simulink model "hw2_eserc_4_simulink_new"  (R2023b)
settings: Solver=FixedStepAuto  StartTime=0.0  StopTime=10  FixedStep=1/fs  RelTol=1e-3
undefined symbols (not defined in the file or in its folder): b, k1, k2
libraries: robotmobilelib x1
settings Model: Creator=ANDREA  LastModifiedBy=lalla

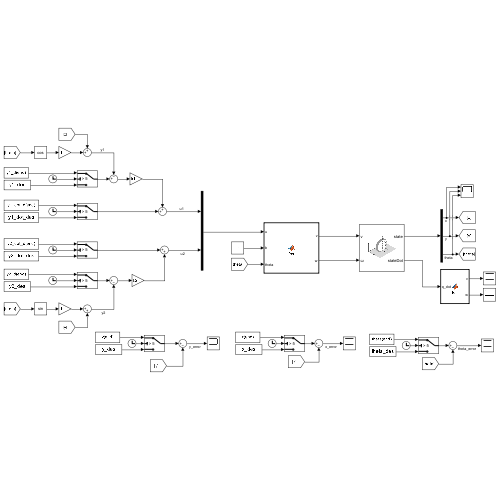
[thumbnail: Simulink's stored preview of the top-level diagram]
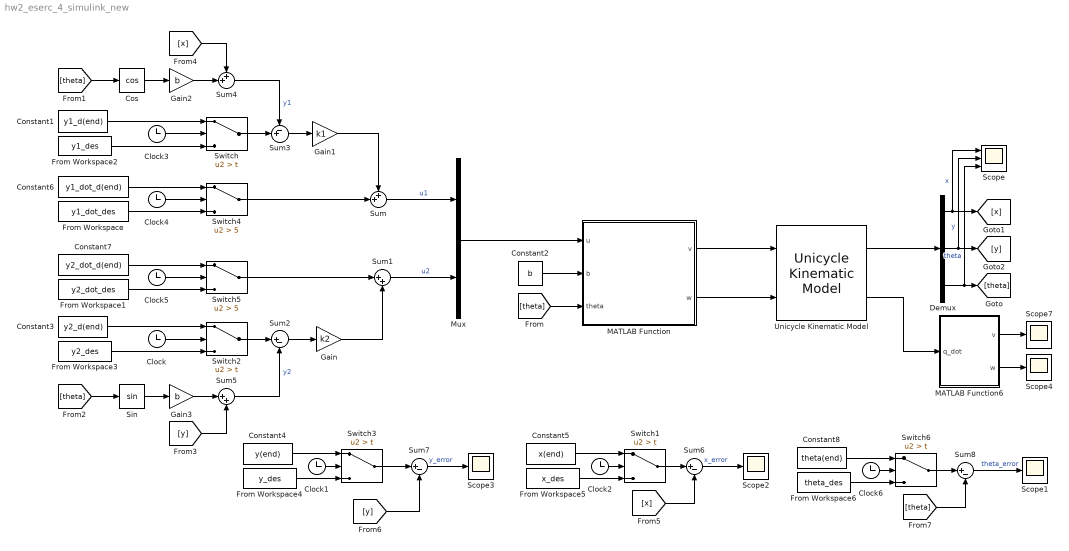
== system hw2_eserc_4_simulink_new ==
  Clock{,1..6} (7 alike) : Clock
  Constant1 : Constant  Value=y1_d(end)
  Constant2 : Constant  Value=b
  Constant3 : Constant  Value=y2_d(end)
  Constant4 : Constant  Value=y(end)
  Constant5 : Constant  Value=x(end)
  Constant6 : Constant  Value=y1_dot_d(end)
  Constant7 : Constant  Value=y2_dot_d(end)
  Constant8 : Constant  Value=theta(end)
  Cos : Trigonometry  Operator=cos
  Demux : Demux  Outputs=3
  From Workspace : FromWorkspace  VariableName=y1_dot_des
  From Workspace1 : FromWorkspace  VariableName=y2_dot_des
  From Workspace2 : FromWorkspace  VariableName=y1_des
  From Workspace3 : FromWorkspace  VariableName=y2_des
  From Workspace4 : FromWorkspace  VariableName=y_des
  From Workspace5 : FromWorkspace  VariableName=x_des
  From Workspace6 : FromWorkspace  VariableName=theta_des
  Gain : Gain  Gain=k2
  Gain1 : Gain  Gain=k1
  Gain2 : Gain  Gain=b
  Gain3 : Gain  Gain=b
  MATLAB Function : MATLAB Function  TreatAsAtomicUnit=on
  MATLAB Function6 : MATLAB Function  TreatAsAtomicUnit=on
  Mux : Mux  Inputs=2
  Scope : Scope  NumInputPorts=3
  Scope{1..4,7} (5 alike) : Scope
  Sin : Trigonometry
  Sum : Sum  Inputs=++|
  Sum1 : Sum  Inputs=|++
  Sum{2,6..8} (4 alike) : Sum  Inputs=|+-
  Sum3 : Sum  Inputs=-+|
  Sum4 : Sum  Inputs=++|
  Sum5 : Sum  Inputs=|++
  Switch{,1..3,6} (5 alike) : Switch  Criteria=u2 > Threshold  Threshold=t  SaturateOnIntegerOverflow=off  InputSameDT=off
  Switch4 : Switch  Criteria=u2 > Threshold  Threshold=5  SaturateOnIntegerOverflow=off  InputSameDT=off
  Switch5 : Switch  Criteria=u2 > Threshold  Threshold=5  SaturateOnIntegerOverflow=off  InputSameDT=off
  Unicycle Kinematic Model : robotmobilelib/Unicycle Kinematic Model  VehicleInputs=Vehicle Speed & Heading Angular Velocity  WheelRadius=b  WheelSpeedRange=[-Inf Inf]  InitialState=[0; 0; 0]  SimulateUsing=Interpreted execution
  wires:
  Unicycle Kinematic Model/1 -> Demux/1
  Gain/1 -> Sum1/2
  Sum3/1 -> Gain1/1
  Sum2/1 -> Gain/1
  Constant2/1 -> MATLAB Function/2(b)
  Cos/1 -> Gain2/1
  Sin/1 -> Gain3/1
  Demux/3 -> Scope/3, [theta]  "theta"
  [theta] -> MATLAB Function/3(theta)
  [theta] -> Cos/1
  [theta] -> Sin/1
  Gain2/1 -> Sum4/2
  Sum/1 -> Mux/1  "u1"
  Sum1/1 -> Mux/2  "u2"
  Mux/1 -> MATLAB Function/1(u)
  Demux/1 -> Scope/1, [x]  "x"
  Demux/2 -> Scope/2, [y]  "y"
  [x] -> Sum4/1
  Gain3/1 -> Sum5/1
  [y] -> Sum5/2
  MATLAB Function/2(w) -> Unicycle Kinematic Model/2
  MATLAB Function/1(v) -> Unicycle Kinematic Model/1
  Sum7/1 -> Scope3/1  "y_error"
  Sum6/1 -> Scope2/1  "x_error"
  Gain1/1 -> Sum/1
  Sum5/1 -> Sum2/2  "y2"
  Sum4/1 -> Sum3/1  "y1"
  [y] -> Sum7/2
  [x] -> Sum6/2
  Switch2/1 -> Sum2/1
  Clock/1 -> Switch2/2
  Switch3/1 -> Sum7/1
  Switch1/1 -> Sum6/1
  Clock2/1 -> Switch1/2
  Switch/1 -> Sum3/2
  Clock3/1 -> Switch/2
  Clock1/1 -> Switch3/2
  Clock4/1 -> Switch4/2
  Switch4/1 -> Sum/2
  Clock5/1 -> Switch5/2
  Switch5/1 -> Sum1/1
  Constant1/1 -> Switch/1
  From Workspace2/1 -> Switch/3
  Constant3/1 -> Switch2/1
  From Workspace3/1 -> Switch2/3
  From Workspace1/1 -> Switch5/3
  Constant7/1 -> Switch5/1
  Constant6/1 -> Switch4/1
  From Workspace/1 -> Switch4/3
  From Workspace4/1 -> Switch3/3
  Constant4/1 -> Switch3/1
  From Workspace5/1 -> Switch1/3
  Constant5/1 -> Switch1/1
  MATLAB Function6/1(v) -> Scope7/1
  Unicycle Kinematic Model/2 -> MATLAB Function6/1(q_dot)
  MATLAB Function6/2(w) -> Scope4/1
  From Workspace6/1 -> Switch6/3
  Sum8/1 -> Scope1/1  "theta_error"
  Constant8/1 -> Switch6/1
  [theta] -> Sum8/2
  Clock6/1 -> Switch6/2
  Switch6/1 -> Sum8/1

== matlab function hw2_eserc_4_simulink_new/MATLAB Function ==
  data: u input; b input; theta input; v output; w output
function [v,w] = fcn(u, b, theta)
T = [cos(theta) -b*sin(theta);
     sin(theta) b*cos(theta)];
sol = inv(T)*u;
v = sol(1);
w = sol(2);

== matlab function hw2_eserc_4_simulink_new/MATLAB Function6 ==
  data: q_dot input; v output; w output
function [v,w] = fcn(q_dot)
v= sqrt(q_dot(1)^2 + q_dot(2)^2);
w= q_dot(3);
